simulink model "ZN_cl_comparison_weighted_s"  (R2021b)
settings: Solver=VariableStepAuto  StartTime=0.0  StopTime=15  RelTol=1e-3
settings Model: Creator=nima8  LastModifiedBy=nima8

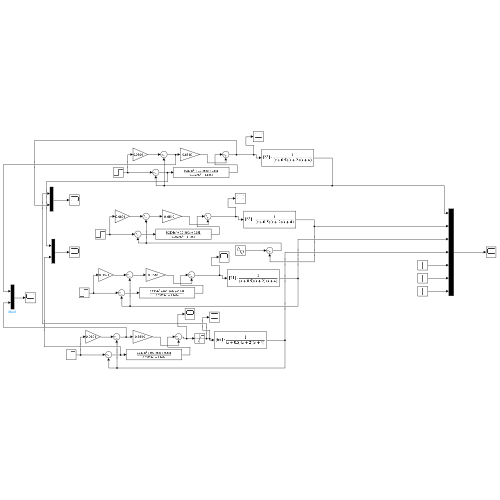
[thumbnail: Simulink's stored preview of the top-level diagram]
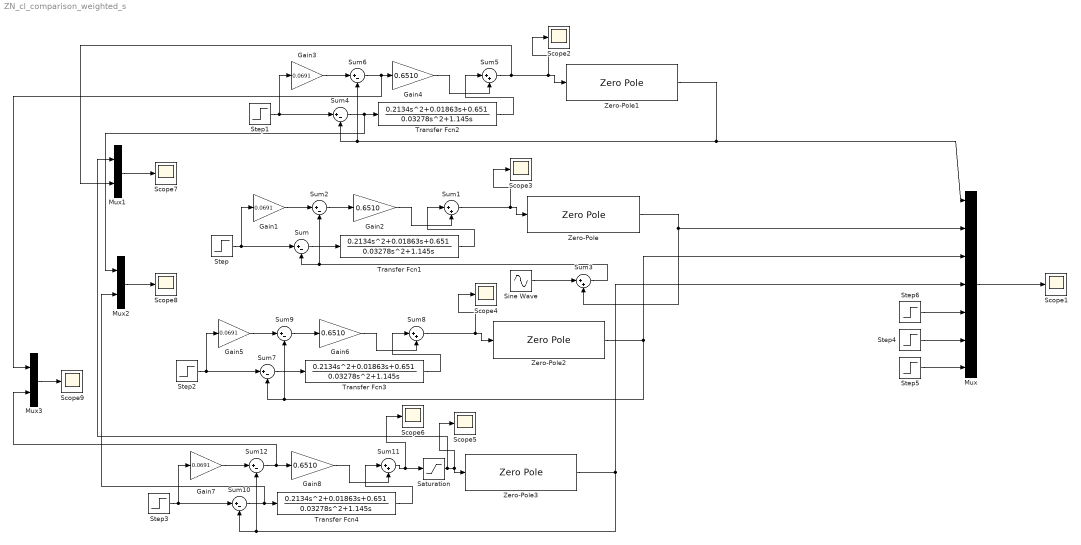
== system ZN_cl_comparison_weighted_s ==
  Gain{1,3,5,7} (4 alike) : Gain  Gain=0.0691
  Gain{2,4,6,8} (4 alike) : Gain  Gain=0.6510
  Mux : Mux  Inputs=7
  Mux1 : Mux  Inputs=2
  Mux2 : Mux  Inputs=2
  Mux3 : Mux  Inputs=2
  Saturation : Saturate  UpperLimit=4.55  LowerLimit=0.1
  Scope{1..9} (9 alike) : Scope
  Sine Wave : Sin  Amplitude=0.1  Frequency=60  SampleTime=0
  Step{,1..3,6} (5 alike) : Step  Time=0  SampleTime=0
  Step4 : Step  Time=0  After=0.98  SampleTime=0
  Step5 : Step  Time=0  After=1.02  SampleTime=0
  Sum{,2,4,6..7,9..10,12} (8 alike) : Sum  Inputs=|+-
  Sum{1,3,5,8,11} (5 alike) : Sum  Inputs=|++
  Transfer Fcn{1..4} (4 alike) : TransferFcn  Numerator=[0.2134 0.01863 0.651]  Denominator=[0.03278 1.145 0]
  Zero-Pole : ZeroPole  Zeros=[]  Poles=[-0.5 -2 -4]  Gain=[63]
  Zero-Pole1 : ZeroPole  Zeros=[]  Poles=[-0.5 -2 -4]  Gain=[63]
  Zero-Pole2 : ZeroPole  Zeros=[]  Poles=[-0.5 -2 -4]  Gain=[21]
  Zero-Pole3 : ZeroPole  Zeros=[]  Poles=[-0.5 -2 -4]  Gain=[63]
  wires:
  Mux/1 -> Scope1/1
  Step4/1 -> Mux/6
  Step5/1 -> Mux/7
  Step6/1 -> Mux/5
  Gain1/1 -> Sum2/1
  Sum/1 -> Transfer Fcn1/1
  Sum3/1 -> Sum2/2, Sum/2
  Gain2/1 -> Sum1/2
  Sum1/1 -> Scope3/1, Zero-Pole/1
  Sum2/1 -> Gain2/1
  Zero-Pole/1 -> Mux/2, Sum3/2
  Transfer Fcn1/1 -> Sum1/1
  Step/1 -> Gain1/1, Sum/1
  Sine Wave/1 -> Sum3/1
  Sum5/1 -> Mux1/2, Scope2/1, Zero-Pole1/1
  Gain4/1 -> Sum5/2
  Sum4/1 -> Mux2/1, Transfer Fcn2/1
  Transfer Fcn2/1 -> Sum5/1
  Gain3/1 -> Sum6/1
  Step1/1 -> Gain3/1, Sum4/1
  Sum6/1 -> Mux3/1, Gain4/1
  Zero-Pole1/1 -> Mux/1, Sum6/2, Sum4/2
  Step2/1 -> Gain5/1, Sum7/1
  Sum9/1 -> Gain6/1
  Gain5/1 -> Sum9/1
  Gain6/1 -> Sum8/2
  Zero-Pole2/1 -> Sum9/2, Sum7/2, Mux/3
  Sum8/1 -> Scope4/1, Zero-Pole2/1
  Sum7/1 -> Transfer Fcn3/1
  Transfer Fcn3/1 -> Sum8/1
  Step3/1 -> Gain7/1, Sum10/1
  Sum12/1 -> Mux3/2, Gain8/1
  Gain7/1 -> Sum12/1
  Gain8/1 -> Sum11/2
  Zero-Pole3/1 -> Sum12/2, Sum10/2, Mux/4
  Sum10/1 -> Mux2/2, Transfer Fcn4/1
  Transfer Fcn4/1 -> Sum11/1
  Saturation/1 -> Scope5/1, Zero-Pole3/1, Mux1/1
  Sum11/1 -> Scope6/1, Saturation/1
  Mux1/1 -> Scope7/1
  Mux2/1 -> Scope8/1
  Mux3/1 -> Scope9/1
